simulink model "finalhw8"  (R2019a)
settings: Solver=VariableStepAuto  StartTime=0.0  StopTime=1  RelTol=1e-3
settings Model: Creator=sumli  LastModifiedBy=sumli

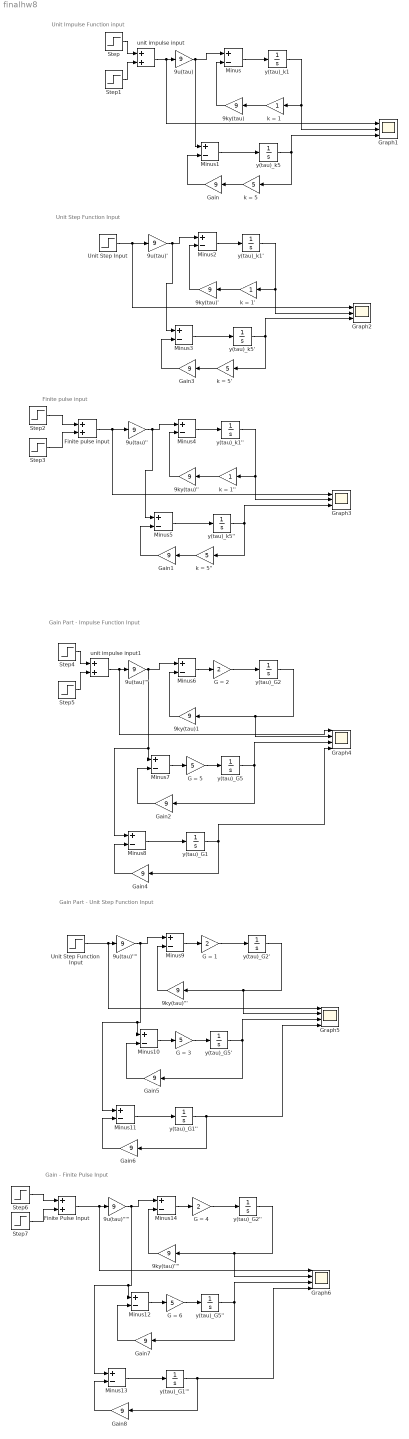
== system finalhw8 ==
  note: Gain - Finite Pulse Input
  note: Gain Part - Unit Step Function Input
  note: Gain Part - Impulse Function Input
  note: Finite pulse input
  note: Unit Step Function Input
  note: Unit Impulse Function input
  9ky(tau) : Gain  Gain=9
  9ky(tau)' : Gain  Gain=9
  9ky(tau)'' : Gain  Gain=9
  9ky(tau)''' : Gain  Gain=9
  9ky(tau)'''' : Gain  Gain=9
  9ky(tau)1 : Gain  Gain=9
  9u(tau) : Gain  Gain=9
  9u(tau)' : Gain  Gain=9
  9u(tau)'' : Gain  Gain=9
  9u(tau)''' : Gain  Gain=9
  9u(tau)'''' : Gain  Gain=9
  9u(tau)''''' : Gain  Gain=9
  Finite Pulse Input : Sum
  Finite pulse input : Sum
  G = 1 : Gain  Gain=2
  G = 2 : Gain  Gain=2
  G = 3 : Gain  Gain=5
  G = 4 : Gain  Gain=2
  G = 5 : Gain  Gain=5
  G = 6 : Gain  Gain=5
  Gain{,1..8} (9 alike) : Gain  Gain=9
  Graph1 : Scope  NumInputPorts=3
  Graph2 : Scope  NumInputPorts=3
  Graph3 : Scope  NumInputPorts=3
  Graph4 : Scope  NumInputPorts=4
  Graph5 : Scope  NumInputPorts=4
  Graph6 : Scope  NumInputPorts=4
  Minus{,1..14} (15 alike) : Sum  Inputs=+-
  Step : Step  Time=0  After=10000  SampleTime=0
  Step1 : Step  Time=0.0001  After=-10000  SampleTime=0
  Step2 : Step  Time=0  SampleTime=0
  Step3 : Step  Time=1/9  After=-1  SampleTime=0
  Step4 : Step  Time=0  After=10000  SampleTime=0
  Step5 : Step  Time=0.0001  After=-10000  SampleTime=0
  Step6 : Step  Time=0  SampleTime=0
  Step7 : Step  Time=1/9  After=-1  SampleTime=0
  Unit Step Function Input : Step  Time=0  SampleTime=0
  Unit Step Input : Step  Time=0  SampleTime=0
  k = 1 : Gain
  k = 1' : Gain
  k = 1'' : Gain
  k = 5 : Gain  Gain=5
  k = 5' : Gain  Gain=5
  k = 5'' : Gain  Gain=5
  unit impulse input : Sum
  unit impulse input1 : Sum
  y(tau)_G1 : Integrator
  y(tau)_G1'' : Integrator
  y(tau)_G1''' : Integrator
  y(tau)_G2 : Integrator
  y(tau)_G2' : Integrator
  y(tau)_G2'' : Integrator
  y(tau)_G5 : Integrator
  y(tau)_G5' : Integrator
  y(tau)_G5'' : Integrator
  y(tau)_k1 : Integrator
  y(tau)_k1' : Integrator
  y(tau)_k1'' : Integrator
  y(tau)_k5 : Integrator
  y(tau)_k5' : Integrator
  y(tau)_k5'' : Integrator
  wires:
  Step/1 -> unit impulse input/1
  Step1/1 -> unit impulse input/2
  unit impulse input/1 -> Graph1/1, 9u(tau)/1
  9u(tau)/1 -> Minus1/1, Minus/1
  Minus/1 -> y(tau)_k1/1
  k = 1/1 -> 9ky(tau)/1
  9ky(tau)/1 -> Minus/2
  y(tau)_k1/1 -> Graph1/2, k = 1/1
  Minus1/1 -> y(tau)_k5/1
  y(tau)_k5/1 -> Graph1/3, k = 5/1
  k = 5/1 -> Gain/1
  Gain/1 -> Minus1/2
  Unit Step Input/1 -> Graph2/1, 9u(tau)'/1
  Minus2/1 -> y(tau)_k1'/1
  9u(tau)'/1 -> Minus3/1, Minus2/1
  k = 1'/1 -> 9ky(tau)'/1
  9ky(tau)'/1 -> Minus2/2
  Minus3/1 -> y(tau)_k5'/1
  y(tau)_k1'/1 -> Graph2/2, k = 1'/1
  Gain3/1 -> Minus3/2
  y(tau)_k5'/1 -> Graph2/3, k = 5'/1
  k = 5'/1 -> Gain3/1
  Finite pulse input/1 -> Graph3/1, 9u(tau)''/1
  9ky(tau)''/1 -> Minus4/2
  k = 1''/1 -> 9ky(tau)''/1
  y(tau)_k5''/1 -> Graph3/3, k = 5''/1
  Minus4/1 -> y(tau)_k1''/1
  9u(tau)''/1 -> Minus5/1, Minus4/1
  Minus5/1 -> y(tau)_k5''/1
  k = 5''/1 -> Gain1/1
  Gain1/1 -> Minus5/2
  y(tau)_k1''/1 -> Graph3/2, k = 1''/1
  Step2/1 -> Finite pulse input/1
  Step3/1 -> Finite pulse input/2
  Step4/1 -> unit impulse input1/1
  unit impulse input1/1 -> Graph4/1, 9u(tau)'''/1
  y(tau)_G5/1 -> Graph4/3, Gain2/1
  y(tau)_G2/1 -> 9ky(tau)1/1, Graph4/2
  9ky(tau)1/1 -> Minus6/2
  Step5/1 -> unit impulse input1/2
  Gain2/1 -> Minus7/2
  Gain4/1 -> Minus8/2
  9u(tau)'''/1 -> Minus8/1, Minus7/1, Minus6/1
  y(tau)_G1/1 -> Graph4/4, Gain4/1
  Minus8/1 -> y(tau)_G1/1
  Minus6/1 -> G = 2/1
  G = 2/1 -> y(tau)_G2/1
  Minus7/1 -> G = 5/1
  G = 5/1 -> y(tau)_G5/1
  Minus11/1 -> y(tau)_G1''/1
  9ky(tau)'''/1 -> Minus9/2
  G = 1/1 -> y(tau)_G2'/1
  Unit Step Function Input/1 -> Graph5/1, 9u(tau)''''/1
  G = 3/1 -> y(tau)_G5'/1
  Gain6/1 -> Minus11/2
  Minus9/1 -> G = 1/1
  y(tau)_G1''/1 -> Graph5/4, Gain6/1
  Gain5/1 -> Minus10/2
  y(tau)_G5'/1 -> Graph5/3, Gain5/1
  9u(tau)''''/1 -> Minus11/1, Minus10/1, Minus9/1
  y(tau)_G2'/1 -> 9ky(tau)'''/1, Graph5/2
  Minus10/1 -> G = 3/1
  y(tau)_G2''/1 -> 9ky(tau)''''/1, Graph6/2
  y(tau)_G5''/1 -> Graph6/3, Gain7/1
  9ky(tau)''''/1 -> Minus14/2
  Minus13/1 -> y(tau)_G1'''/1
  Gain8/1 -> Minus13/2
  y(tau)_G1'''/1 -> Graph6/4, Gain8/1
  Gain7/1 -> Minus12/2
  G = 4/1 -> y(tau)_G2''/1
  G = 6/1 -> y(tau)_G5''/1
  9u(tau)'''''/1 -> Minus13/1, Minus12/1, Minus14/1
  Minus12/1 -> G = 6/1
  Minus14/1 -> G = 4/1
  Finite Pulse Input/1 -> Graph6/1, 9u(tau)'''''/1
  Step6/1 -> Finite Pulse Input/1
  Step7/1 -> Finite Pulse Input/2
